simulink model "VTOL_sim"  (R2016b)
settings: Solver=ode45  StartTime=0.0  StopTime=100  RelTol=1e-3  EnableMultiTasking=on
InitFcn:
  | addpath ./..
  | VTOL_param
  | VTOLParamHW13
undefined symbols (not defined in the file or in its folder): P, VTOL_animation, VTOL_ctrl
settings Model: Creator=beard  LastModifiedBy=beard
settings DataIOCC: LimitDataPoints=on  SaveFormat=Array  SignalLoggingSaveFormat=ModelDataLogs
settings OptimizationCC: ExpressionDepthLimit=2147483647  InitFltsAndDblsToZero=on  LifeSpan=inf
settings DebuggingCC: UnderspecifiedInitializationDetection=Classic  MergeDetectMultiDrivingBlocksExec=none  SolverPrmCheckMsg=warning  FcnCallInpInsideContextMsg=warning  StateNameClashWarn=warning  SFUnexpectedBacktrackingDiag=warning  SFNoUnconditionalDefaultTransitionDiag=warning  SFExecutionAtInitializationDiag=none
settings HardwareCC: ProdBitPerPointer=32  ProdBitPerSizeT=32  ProdBitPerPtrDiffT=32  ProdLargestAtomicFloat=None  ProdIntDivRoundTo=Undefined  ProdEndianess=Unspecified  ProdWordSize=32  ProdHWDeviceType=32-bit Generic
settings ModelReferenceCC: PropagateSignalLabelsOutOfModel=off
settings GRTTargetCC: TargetLangStandard=C89/C90 (ANSI)  GeneratePreprocessorConditionals=Disable all  CombineOutputUpdateFcns=off  GRTInterface=on
settings ConfigComp: CovMetricSettings=dw  CovHtmlReporting=on  CovSaveCumulativeToWorkspaceVar=on  CovSaveSingleToWorkspaceVar=on  CovExternalEMLEnable=off

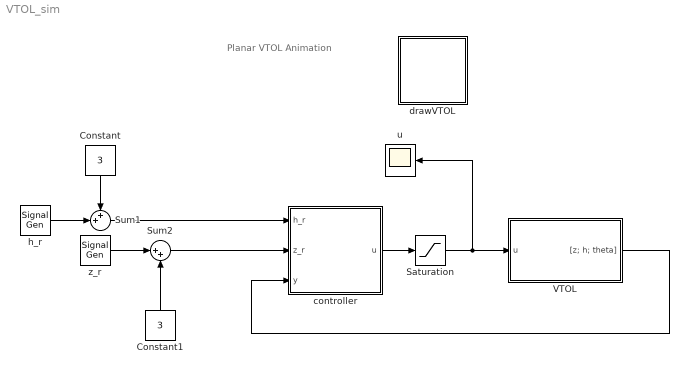
== system VTOL_sim ==
  note: Planar VTOL Animation
  Constant : Constant  Value=3
  Constant1 : Constant  Value=3
  Saturation : Saturate  UpperLimit=P.fmax  LowerLimit=0
  Sum1 : Sum  Inputs=++|
  Sum2 : Sum  Inputs=|++
  VTOL : Subsystem
  controller : Subsystem
  drawVTOL : Subsystem
      mask Display: image(imread('tv.jpg'))
  h_r : SignalGenerator  WaveForm=square  Amplitude=2.5  Frequency=.03
  u : Scope
  z_r : SignalGenerator  WaveForm=square  Amplitude=2.5  Frequency=.02
  wires:
  Constant/1 -> Sum1/1
  h_r/1 -> Sum1/2
  Sum2/1 -> controller/2(z_r)
  z_r/1 -> Sum2/1
  Constant1/1 -> Sum2/2
  Saturation/1 -> VTOL/1(u), u/1
  controller/1(u) -> Saturation/1
  Sum1/1 -> controller/1(h_r)
  VTOL/1("[z; h; theta]") -> controller/3(y)

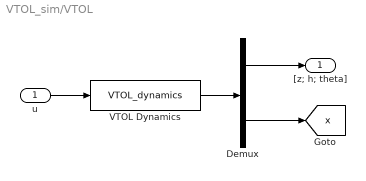
== system VTOL_sim/VTOL ==
  u : Inport
  Demux : Demux  Outputs=[3;6]
  VTOL Dynamics : S-Function  FunctionName=VTOL_dynamics  Parameters=P  SFunctionDeploymentMode=off  EnableBusSupport=off
  "[z; h; theta]" : Outport
  tag scope: x=global
  wires:
  Demux/2 -> [x]
  Demux/1 -> "[z; h; theta]"/1
  VTOL Dynamics/1 -> Demux/1
  u/1 -> VTOL Dynamics/1

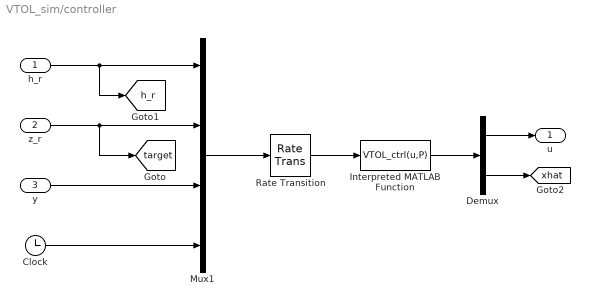
== system VTOL_sim/controller ==
  h_r : Inport
  z_r : Inport  Port=2
  y : Inport  Port=3
  Clock : Clock
  Demux : Demux  Outputs=[2;6]
  Interpreted MATLAB Function : MATLABFcn  MATLABFcn=VTOL_ctrl(u,P)  OutputDimensions=2+6
  Mux1 : Mux
  Rate Transition : RateTransition  OutPortSampleTime=P.Ts
  u : Outport
  tag scope: h_r=global, target=global, xhat=global
  wires:
  Mux1/1 -> Rate Transition/1
  h_r/1 -> [h_r], Mux1/1
  Clock/1 -> Mux1/4
  Rate Transition/1 -> Interpreted MATLAB Function/1
  y/1 -> Mux1/3
  z_r/1 -> [target], Mux1/2
  Interpreted MATLAB Function/1 -> Demux/1
  Demux/1 -> u/1
  Demux/2 -> [xhat]

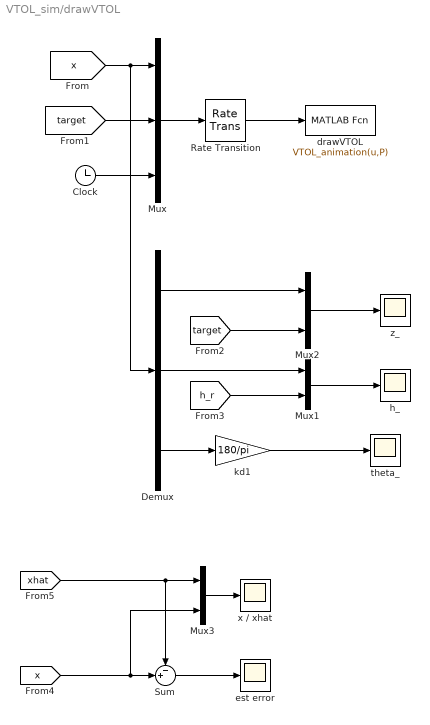
== system VTOL_sim/drawVTOL ==
  Clock : Clock
  Demux : Demux  Outputs=3
  Mux : Mux  Inputs=3
  Mux1 : Mux  Inputs=2
  Mux2 : Mux  Inputs=2
  Mux3 : Mux  Inputs=2
  Rate Transition : RateTransition  OutPortSampleTime=P.t_plot
  Sum : Sum  Inputs=-+|
  drawVTOL : MATLABFcn  MATLABFcn=VTOL_animation(u,P)  OutputDimensions=0
  est error : Scope
  h_ : Scope
  kd1 : Gain  Gain=180/pi
  theta_ : Scope
  x / xhat : Scope
  z_ : Scope
  wires:
  [x] -> Sum/2, Mux3/2
  [xhat] -> Sum/1, Mux3/1
  Sum/1 -> est error/1
  Mux3/1 -> x / xhat/1
  [h_r] -> Mux1/2
  Demux/2 -> Mux1/1
  [target] -> Mux2/2
  Demux/1 -> Mux2/1
  Demux/3 -> kd1/1
  kd1/1 -> theta_/1
  Mux2/1 -> z_/1
  Mux1/1 -> h_/1
  [x] -> Mux/1, Demux/1
  Mux/1 -> Rate Transition/1
  Clock/1 -> Mux/3
  Rate Transition/1 -> drawVTOL/1
  [target] -> Mux/2
